simulink model "hipotenso"  (R2024b)
settings: Solver=ode15s  StartTime=0.0  StopTime=10.0  MaxStep=1e-3  RelTol=1e-3
libraries: slpidlib x1
settings Model: LastModifiedBy=Panzzi
settings DataIOCC: ReturnWorkspaceOutputs=off  TimeSaveName=t
settings DebuggingCC: AlgebraicLoopMsg=none  ArtificialAlgebraicLoopMsg=none  SaveWithDisabledLinksMsg=none  SaveWithParameterizedLinksMsg=none  BlockPriorityViolationMsg=error  MinStepSizeMsg=error  MaxConsecutiveZCsMsg=none  MaskedZcDiagnostic=none  IgnoredZcDiagnostic=none  ModelReferenceSymbolNameMessage=none  OperatingPointInterfaceChecksumMismatchMsg=none  InitInArrayFormatMsg=none  UnitsInconsistencyMsg=none

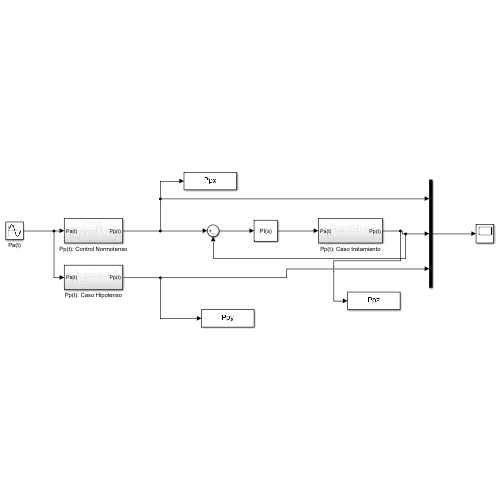
[thumbnail: Simulink's stored preview of the top-level diagram]
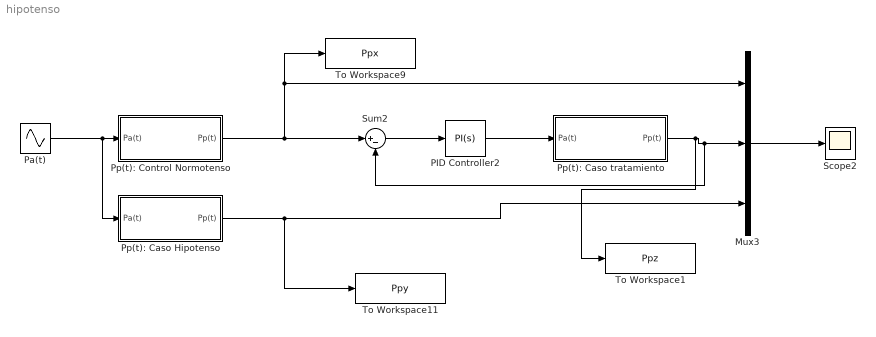
== system hipotenso ==
  Mux3 : Mux  Inputs=3
  PID Controller2 : slpidlib/PID Controller  Controller=PI  Form=Parallel  TimeDomain=Continuous-time  UseExternalTs=off  SampleTime=-1  IntegratorMethod=Forward Euler  FilterMethod=Forward Euler  ControllerParametersSource=internal  P=0.00206  I=10333.33  UseKiTs=off  D=0  UseExternalDerivativeSource=off  N=100  UseFilter=on  TunerSelectOption=Transfer Function Based (PID Tuner App)  InitialConditionSource=internal  InitialConditionForIntegrator=0  InitialConditionForFilter=0  DifferentiatorICPrevScaledInput=0  ExternalReset=none  TrackingMode=off  Kt=1  LimitOutput=off  SatLimitsSource=internal  UpperSaturationLimit=inf  LowerSaturationLimit=-inf  LinearizeAsGain=on  AntiWindupMode=none  Kb=1  LimitIntegrator=off  UpperIntegratorSaturationLimit=inf  LowerIntegratorSaturationLimit=-inf  POutMin=[]  POutMax=[]  IOutMin=[]  IOutMax=[]  DOutMin=[]  DOutMax=[]  NOutMin=[]  NOutMax=[]  SumOutMin=[]  SumOutMax=[]  SaturationOutMin=[]  SaturationOutMax=[]  PParamMin=[]  PParamMax=[]  IParamMin=[]  IParamMax=[]  DParamMin=[]  DParamMax=[]  NParamMin=[]  NParamMax=[]  KbParamMin=[]  KbParamMax=[]  KtParamMin=[]  KtParamMax=[]  KbOutMin=[]  KbOutMax=[]  KtOutMin=[]  KtOutMax=[]  IntegratorOutMin=[]  IntegratorOutMax=[]  FilterOutMin=[]  FilterOutMax=[]  SumI1OutMin=[]  SumI1OutMax=[]  SumI2OutMin=[]  SumI2OutMax=[]  SumI3OutMin=[]  SumI3OutMax=[]  SumI4OutMin=[]  SumI4OutMax=[]  SumDOutMin=[]  SumDOutMax=[]  DifferentiatorOutMin=[]  DifferentiatorOutMax=[]  FilterDiffOutCoefMin=[]  FilterDiffOutCoefMax=[]  ReciprocalOutMin=[]  ReciprocalOutMax=[]  SumDenOutMin=[]  SumDenOutMax=[]  SumNumOutMin=[]  SumNumOutMax=[]  DivideOutMin=[]  DivideOutMax=[]  UdiffTsProdOutMin=[]  UdiffTsProdOutMax=[]  NTsProdOutMin=[]  NTsProdOutMax=[]  UintegralTsProdOutMin=[]  UintegralTsProdOutMax=[]  UngainTsProdOutMin=[]  UngainTsProdOutMax=[]  ClampingZeroOutDataTypeStr=Inherit: Inherit via back propagation  ClampingZeroOutMin=[]  ClampingZeroOutMax=[]  FilterDenConstantOutDataTypeStr=Inherit: Inherit via back propagation  FilterDenConstantOutMin=[]  FilterDenConstantOutMax=[]  PCopyOutDataTypeStr=Inherit: Inherit via back propagation  PCopyOutMin=[]  PCopyOutMax=[]  NCopyOutDataTypeStr=Inherit: Inherit via back propagation  NCopyOutMin=[]  NCopyOutMax=[]  IntegratorContinuousStateAttributes=''  IntegratorStateMustResolveToSignalObject=off  IntegratorRTWStateStorageClass=Auto  FilterContinuousStateAttributes=''  FilterStateMustResolveToSignalObject=off  FilterRTWStateStorageClass=Auto  ParallelPVariant=InternalParameters  IdealPVariant=Disabled  IVariant=InternalParameters  DVariant=Disabled  IntegratorVariant=Continuous  SatVariant=Disabled  AWVariant=Passthrough  PCopyVariant=Disabled  TRVariant=Disabled  FdbkBlocksVariant=Forward  IdealPFdbkVariant=Disabled  SatFdbkVariant=Disabled  DerivativeFilterVariant=Disabled  NVariant=Disabled  NCopyVariant=Disabled_SignalSpec  FilterICVariant=Disabled  IntegratorICVariant=InternalICs  ExternalResetVariant=Disabled  TRSumVariant=Passthrough  SumFdbkVariant=Disabled  SumVariant=Sum_PI  TsampFilterVariant=InternalTs  TsampNgainVariant=Passthrough  TsampIntegralVariant=Disabled_SignalSpec  ExternalSaturationOutDataTypeStr=Inherit: Same as second input  DerivativeSourceVariant=Disabled  PreIntVariant=InternalPreInt
  Pa(t) : Sin  Bias=0.8  Frequency=2*pi*95/60  SampleTime=0
  Pp(t): Caso Hipotenso : Subsystem
  Pp(t): Caso tratamiento : Subsystem
  Pp(t): Control Normotenso : Subsystem
  Scope2 : Scope
  Sum2 : Sum  Inputs=|+-
  To Workspace1 : ToWorkspace  VariableName=Ppz  SampleTime=-1
  To Workspace11 : ToWorkspace  VariableName=Ppy  SampleTime=-1
  To Workspace9 : ToWorkspace  VariableName=Ppx  SampleTime=-1
  wires:
  Pa(t)/1 -> Pp(t): Caso Hipotenso/1(Pa(t)), Pp(t): Control Normotenso/1(Pa(t))
  PID Controller2/1 -> Pp(t): Caso tratamiento/1(Pa(t))
  Mux3/1 -> Scope2/1
  Pp(t): Control Normotenso/1(Pp(t)) -> To Workspace9/1, Mux3/1, Sum2/1
  Pp(t): Caso tratamiento/1(Pp(t)) -> To Workspace1/1, Mux3/2, Sum2/2
  Sum2/1 -> PID Controller2/1
  Pp(t): Caso Hipotenso/1(Pp(t)) -> To Workspace11/1, Mux3/3

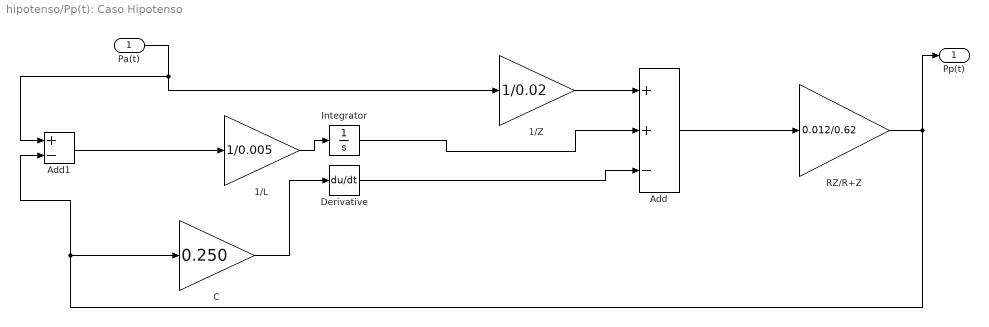
== system hipotenso/Pp(t): Caso Hipotenso ==
  Pa(t) : Inport
  1/L : Gain  Gain=1/0.005
  1/Z : Gain  Gain=1/0.02
  Add : Sum  Inputs=++-
  Add1 : Sum  Inputs=+-
  C : Gain  Gain=0.250
  Derivative : Derivative
  Integrator : Integrator
  RZ/R+Z : Gain  Gain=0.012/0.62
  Pp(t) : Outport
  wires:
  1/Z/1 -> Add/1
  Integrator/1 -> Add/2
  C/1 -> Derivative/1
  RZ/R+Z/1 -> Pp(t)/1, Add1/2, C/1
  Add1/1 -> 1/L/1
  Derivative/1 -> Add/3
  1/L/1 -> Integrator/1
  Pa(t)/1 -> Add1/1, 1/Z/1
  Add/1 -> RZ/R+Z/1

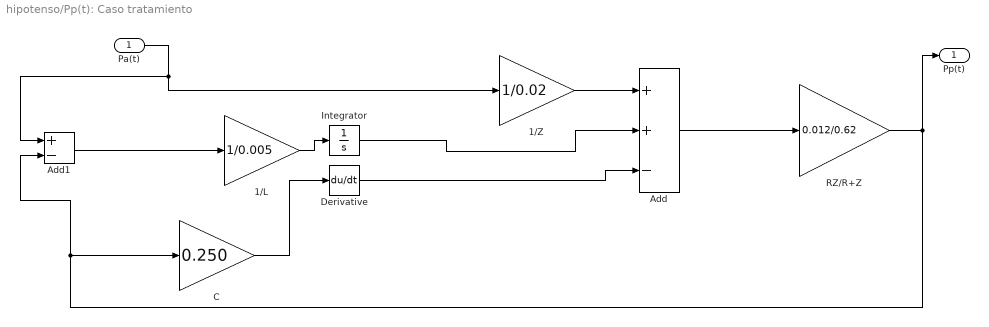
== system hipotenso/Pp(t): Caso tratamiento ==
  Pa(t) : Inport
  1/L : Gain  Gain=1/0.005
  1/Z : Gain  Gain=1/0.02
  Add : Sum  Inputs=++-
  Add1 : Sum  Inputs=+-
  C : Gain  Gain=0.250
  Derivative : Derivative
  Integrator : Integrator
  RZ/R+Z : Gain  Gain=0.012/0.62
  Pp(t) : Outport
  wires:
  1/Z/1 -> Add/1
  Integrator/1 -> Add/2
  C/1 -> Derivative/1
  RZ/R+Z/1 -> Pp(t)/1, Add1/2, C/1
  Add1/1 -> 1/L/1
  Derivative/1 -> Add/3
  1/L/1 -> Integrator/1
  Pa(t)/1 -> Add1/1, 1/Z/1
  Add/1 -> RZ/R+Z/1

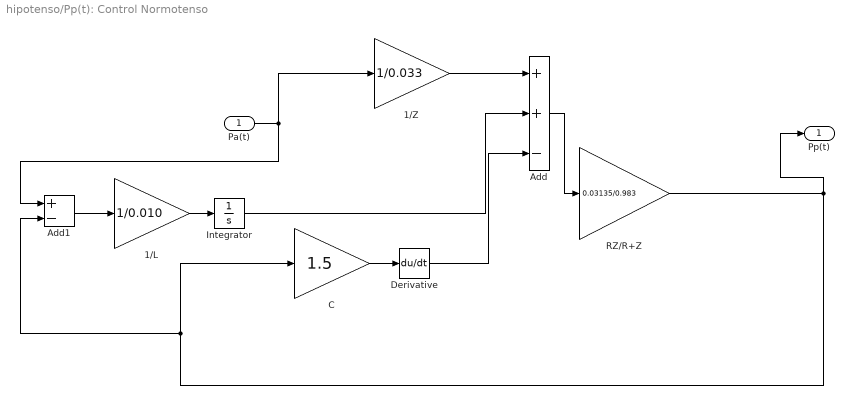
== system hipotenso/Pp(t): Control Normotenso ==
  Pa(t) : Inport
  1/L : Gain  Gain=1/0.010
  1/Z : Gain  Gain=1/0.033
  Add : Sum  Inputs=++-
  Add1 : Sum  Inputs=+-
  C : Gain  Gain=1.5
  Derivative : Derivative
  Integrator : Integrator
  RZ/R+Z : Gain  Gain=0.03135/0.983
  Pp(t) : Outport
  wires:
  Pa(t)/1 -> Add1/1, 1/Z/1
  1/Z/1 -> Add/1
  Integrator/1 -> Add/2
  1/L/1 -> Integrator/1
  Add1/1 -> 1/L/1
  Add/1 -> RZ/R+Z/1
  C/1 -> Derivative/1
  Derivative/1 -> Add/3
  RZ/R+Z/1 -> Pp(t)/1, Add1/2, C/1
